simulink model "queuetest_fourth"  (R2018a)
settings: Solver=VariableStepAuto  StartTime=0.0  StopTime=20.0  RelTol=1e-3
undefined symbols (not defined in the file or in its folder): m, n
libraries: dspbuff3 x1
settings Model: Creator=Michael Girbino  LastModifiedBy=Michael Girbino

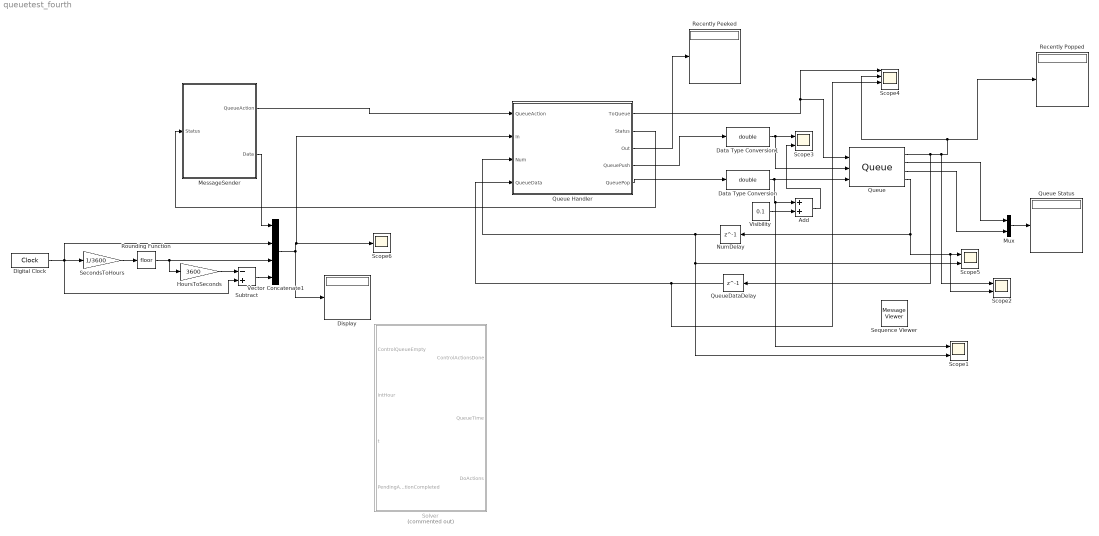
== system queuetest_fourth ==
  Add : Sum
  Data Type Conversion : DataTypeConversion  OutDataTypeStr=double
  Data Type Conversion1 : DataTypeConversion  OutDataTypeStr=double
  Digital Clock : DigitalClock
  Display : Display
  HoursToSeconds : Gain  Gain=3600
  MessageSender : Stateflow chart  TreatAsAtomicUnit=on
  Mux : Mux  Inputs=2
  NumDelay : Delay  DelayLength=1  InitialCondition=0
  Queue : dspbuff3/Queue  depth=10  trigger=Either edge  overflow=Dynamic reallocation  pes=Error  eso=on  fso=on  nso=on  clr=off  clrOutport=off  adf=on
      settings: SourceProductName=DSP System Toolbox  SourceProductBaseCode=DS
  Queue Handler : Stateflow chart  TreatAsAtomicUnit=on
  Queue Status : Display
  QueueDataDelay : Delay  DelayLength=1  InitialCondition=0
  Recently Peeked : Display
  Recently Popped : Display
  Rounding Function : Rounding
  Scope{1..3,5} (4 alike) : Scope  NumInputPorts=2
  Scope4 : Scope  NumInputPorts=4
  Scope6 : Scope
  SecondsToHours : Gain  Gain=1/3600
  Sequence Viewer : MessageViewer
  Solver : Stateflow chart  Commented=on  TreatAsAtomicUnit=on
  Subtract : Sum  Inputs=-+
  Vector Concatenate1 : Concatenate  NumInputs=4
  Visibility : Constant  Value=0.1
  wires:
  Data Type Conversion1/1 -> Scope3/1, Queue/2
  Data Type Conversion/1 -> Scope1/1, Add/1, Queue/3
  Queue Handler/1(ToQueue) -> Scope4/1, Queue/1
  Queue/1 -> QueueDataDelay/1, Scope2/1, Scope4/2, Recently Popped/1
  Queue/3 -> Mux/2
  Queue/2 -> Mux/1
  Mux/1 -> Queue Status/1
  Queue/4 -> NumDelay/1, Scope2/2, Scope5/1
  Queue Handler/4(QueuePush) -> Data Type Conversion1/1
  Queue Handler/5(QueuePop) -> Data Type Conversion/1
  MessageSender/1(QueueAction) -> Queue Handler/1(QueueAction)
  MessageSender/2(Data) -> Vector Concatenate1/1
  Queue Handler/2(Status) -> MessageSender/1(Status)
  NumDelay/1 -> Scope1/2, Scope5/2, Queue Handler/3(Num)
  QueueDataDelay/1 -> Scope4/3, Queue Handler/4(QueueData)
  Queue Handler/3(Out) -> Recently Peeked/1
  Visibility/1 -> Add/2
  Add/1 -> Scope3/2
  Rounding Function/1 -> Vector Concatenate1/3, HoursToSeconds/1
  Digital Clock/1 -> Vector Concatenate1/2, Subtract/2, SecondsToHours/1
  Vector Concatenate1/1 -> Queue Handler/2(In), Scope6/1, Display/1
  SecondsToHours/1 -> Rounding Function/1
  HoursToSeconds/1 -> Subtract/1
  Subtract/1 -> Vector Concatenate1/4

== stateflow chart queuetest_fourth/Solver ==
  (default) -> (junction 25) : % Execute control actions in order based on control mode
  (junction 25) -> (junction 26) [order 1] : [ControlMode == ControlModes.STATIC]
  (junction 26) -> (junction 54)
  (junction 25) -> (junction 29) [order 2]
  (junction 54) -> (junction 55) [order 1] : [ControlQueueEmpty]
      | % execute nearest set of control actions, but leave time where it is
  (junction 54) -> (junction 56) [order 2] : {QueueTime = [0,0]; %xHour, xSec
      | DoActions.data = QueueOps.NearestActions;
      | send(DoActions);
      | % ignores time advancement
      | }
  (junction 55) -> (junction 57) : {ControlActionsDone = true;}
  (junction 57) -> (junction 56)
  (junction 56) -> (junction 27)
  (junction 27) -> (junction 28)
  (junction 28) -> (junction 32)
  (junction 29) -> (junction 30) [order 1] : [ControlMode == ControlModes.EVENTDRIVEN]
      | % execute nearest set of control actions and advance time to that time
  (junction 30) -> (junction 65) : {QueueTime = [intHour,t]; %xHour, xSec
      | DoActions.data = QueueOps.NearestActions;
      | send(DoActions);}
  (junction 29) -> (junction 33) [order 2]
  (junction 65) -> (junction 66) [order 1] : [~PendingActionCompleted]
  (junction 65) -> (junction 67) [order 2]
  (junction 66) -> (junction 68) : {ControlActionsDone = true;
      | % advances time to the next event
      | }
  (junction 68) -> (junction 67)
  (junction 67) -> (junction 31)
  (junction 31) -> (junction 32)
  (junction 32) -> (junction 36)
  (junction 33) -> (junction 34) [order 1] : [ControlMode == ControlModes.TIMEDRIVEN]
      |  % Do all actions having and action time <= specified time
  (junction 34) -> (junction 78) : {QueueTime = [intHour,t]; %xHour, xSec
      | DoActions.data = QueueOps.JustActions;
      | send(DoActions);}
  (junction 33) -> (junction 37) [order 2]
  (junction 78) -> (junction 80) [order 1] : [~PendingActionCompleted]
  (junction 78) -> (junction 79) [order 2]
  (junction 80) -> (junction 82) : {ControlActionsDone = true;
      | }
  (junction 82) -> (junction 79)
  (junction 79) -> (junction 35)
  (junction 35) -> (junction 36)
  (junction 36) -> (junction 40)
  (junction 37) -> (junction 38) [order 1] : [ControlMode == ControlModes.MULTIRATE]
      |  % Execute the nearest set of control actions, but leave time where it is
  (junction 38) -> (junction 91) : {QueueTime = [intHour,t]; %xHour, xSec
      | DoActions.data = QueueOps.MultiRate;
      | send(DoActions);}
  (junction 37) -> (junction 41) [order 2]
  (junction 91) -> (junction 88) [order 1] : [~PendingActionCompleted]
  (junction 91) -> (junction 87) [order 2]
  (junction 88) -> (junction 92) : {ControlActionsDone = true;
      | }
  (junction 92) -> (junction 87)
  (junction 87) -> (junction 39)
  (junction 39) -> (junction 40)
  (junction 40) -> (junction 42)
  (junction 42) -> (junction 41)
  (junction 41) -> (junction 43)
  data: ControlQueueEmpty input boolean; ControlActionsDone output boolean; QueueTime output double size=2; DoActions output double; intHour input uint8; t input uint32; PendingActionCompleted input boolean

== stateflow chart queuetest_fourth/MessageSender ==
  settings: enableNonTerminalStates=1
  state SayPush
    en:
    Data = i;
    QueueAction.data = ...
    QueueActions.PUSH;
    send(QueueAction);
    i = i+1;
  state SayPop
    en:
    QueueAction.data = ...
    QueueActions.POP;
    send(QueueAction);
    i = i+1;
  state SayPeek [commented out]
    en:
    QueueAction.data = 3;
    send(QueueAction);
  state SayPopAgain [commented out]
    en:
    QueueAction.data = 2;
    send(QueueAction);
    i = i+1;
  state Asleep
  (default) -> SayPush : {i = 1;}
  (junction 21) -> SayPush [order 1] : [i <= 9]
  SayPush -> Asleep [order 2] : Status[Status.data == 2]
  SayPush -> (junction 21) [order 1] : Status[Status.data == 1]
  (junction 21) -> SayPop [order 2] : {i = 1;}
  (junction 25) -> SayPop [order 1] : [i <= 9]
  SayPop -> Asleep [order 2] : Status[Status.data == 2]
  SayPop -> (junction 25) [order 1] : Status[Status.data == 1]
  (junction 25) -> Asleep [order 2]
  (junction 25) -> SayPeek [commented out]
  SayPeek -> Asleep [commented out] : Status[Status.data == 2]
  SayPeek -> SayPopAgain [commented out] : Status[Status.data == 1]
  SayPopAgain -> Asleep [commented out] : Status[Status.data == 2]
  (junction 36) -> SayPopAgain [commented out] : [i <= 10]
  SayPopAgain -> (junction 36) [commented out] : Status[Status.data == 1]
  (junction 36) -> Asleep [commented out]
  data: QueueAction output Enum: QueueActions; Data output double; Status input double; i local double

== stateflow chart queuetest_fourth/Queue Handler ==
  settings: enableNonTerminalStates=1
  state Asleep
  state DoNearestActions [commented out]
    (default) -> (junction 117) [commented out] : % do only those actions with the same delay time as the first action time return time
        | {PendingActionsCompleted = false;
        | }
    (junction 117) -> (junction 116) [commented out] : [Num > 0]
    (junction 116) -> (junction 114) [commented out] : {%QueuePeek
        | t = QueueData(1,1); % first item's ActionTime
        | Hour = t.Hour;
        | sec = t.Sec;
        | ii = 2;}
    (junction 117) -> (junction 111) [commented out] : {Status.data = 2;
        | % error
        | send(Status);}
    (junction 114) -> (junction 115) [commented out] : [ii <= Num]
    (junction 115) -> (junction 112) [commented out] : {send(QueuePop);
        | Out = QueueData;
        | %send(DoPendingAction);
        | }
    (junction 112) -> (junction 114) [commented out] : {ii = ii + 1;}
    (junction 114) -> (junction 109) [commented out]
    (junction 109) -> (junction 111) [commented out]
    (junction 111) -> (junction 108) [commented out]
  state Popping
    (default) -> (junction 42)
    (junction 42) -> (junction 52) [order 1] : [Num ~= 0]
    (junction 42) -> (junction 48) [order 2] : {Status.data = 2;
        | % error
        | send(Status);}
    (junction 52) -> (junction 45) : {send(QueuePop);}
    (junction 45) -> (junction 48)
    (junction 48) -> (junction 51)
  state Peeking
    (default) -> (junction 73)
    (junction 73) -> (junction 76) [order 1] : [Num ~= 0]
    (junction 76) -> (junction 65) : {send(QueuePop);
        | Out = QueueData;
        | ToQueue = QueueData;
        | send(QueuePush);
        | }
        | % Put most-recently-viewed data back in front
    (junction 73) -> (junction 78) [order 2] : {Status.data = 2;
        | % error
        | send(Status);}
    (junction 66) -> (junction 64) [order 1] : [ii <= Num]
    (junction 64) -> (junction 67) : {send(QueuePop);
        | ToQueue = QueueData;
        | send(QueuePush);
        | }
    (junction 65) -> (junction 66) : {ii = 2;}
    (junction 67) -> (junction 66) : {ii = ii + 1;}
    (junction 66) -> (junction 70) [order 2]
    (junction 70) -> (junction 78)
    (junction 78) -> (junction 79)
  state DoAllActions
    (default) -> (junction 97)
    (junction 97) -> (junction 100) [order 1] : [Num ~= 0]
    (junction 100) -> (junction 90) : {ii = 2;}
    (junction 97) -> (junction 93) [order 2] : {Status.data = 2;
        | % error
        | send(Status);}
    (junction 90) -> (junction 89) [order 1] : [ii <= Num]
    (junction 89) -> (junction 91) : {send(QueuePop);
        | Out = QueueData;
        | %send(DoPendingAction);
        | }
    (junction 91) -> (junction 90) : {ii = ii + 1;}
    (junction 90) -> (junction 94) [order 2]
    (junction 94) -> (junction 93)
    (junction 93) -> (junction 83)
  state Pushing
    en:
    ToQueue = In;
    send(QueuePush);
  state ReadyAgain
    Status.data = 1; % ready
    send(Status);
  Asleep -> DoNearestActions [commented out] : QueueAction[QueueAction.data == 5]
  (default) -> Asleep
  Asleep -> Popping [order 1] : QueueAction[QueueAction.data == ...
      | QueueActions.POP]
  Asleep -> Pushing [order 2] : QueueAction[QueueAction.data == ...
      | QueueActions.PUSH]
  ReadyAgain -> Asleep
  Asleep -> Peeking [order 3] : QueueAction[QueueAction.data == ...
      | QueueActions.PEEK]
  Asleep -> DoAllActions [order 4] : QueueAction[QueueAction.data == ...
      | QueueActions.DO_ALL_ACTIONS]
  Pushing -> ReadyAgain
  Popping -> ReadyAgain
  DoAllActions -> ReadyAgain
  Peeking -> ReadyAgain
  DoNearestActions -> ReadyAgain [commented out]
  data: QueueAction input Enum: QueueActions; ToQueue output double size=4; In input double size=4; Status output double; Empty local boolean; Num input; NumPops local; QueueData input double; ii local uint8; Out output double size=4
  events: QueuePush output EITHER_EDGE_EVENT; QueuePop output EITHER_EDGE_EVENT
